simulink model "Control_Law_For_Clay"  (R2020b)
settings: Solver=ode45  StartTime=0.0  StopTime=tsim  RelTol=1e-9
undefined symbols (not defined in the file): fric_mod, g_n, Jm, Jp, K, KcRa, Km, L_n, lambda_n, M_n, N_n, switch_law, T_ba_n, x0
libraries: simulink_extras x3, simulink x1
settings Model: Creator=domin  LastModifiedBy=domin
settings SolverCC: ZeroCrossAlgorithm=Adaptive
settings DebuggingCC: IgnoredZcDiagnostic=none

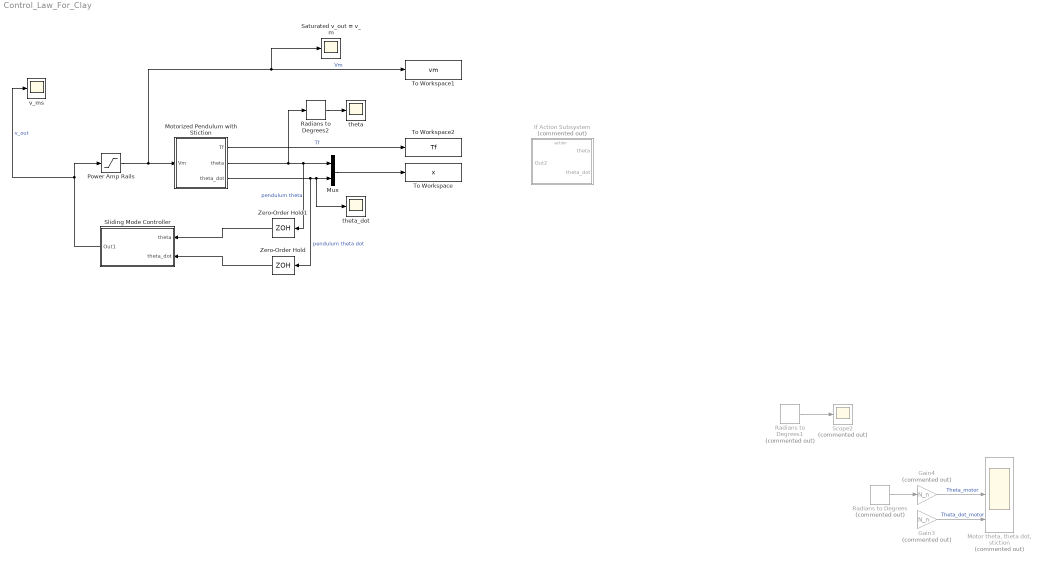
== system Control_Law_For_Clay ==
  Gain3 : Gain  Commented=on  Gain=N_n
  Gain4 : Gain  Commented=on  Gain=N_n
  If Action Subsystem : Subsystem  Commented=on  TreatAsAtomicUnit=on
  "Motor theta, theta dot, stiction" : Scope  Commented=on  NumInputPorts=3
  Motorized Pendulum with Stiction : Subsystem
  Mux : Mux  Inputs=2
  Power Amp Rails : Saturate  UpperLimit=15  LowerLimit=-15
  Radians to Degrees : simulink_extras/Transformations/Radians to Degrees  Commented=on
  Radians to Degrees1 : simulink_extras/Transformations/Radians to Degrees  Commented=on
  Radians to Degrees2 : simulink_extras/Transformations/Radians to Degrees
  Saturated v_out = v_m : Scope
  Scope2 : Scope  Commented=on
  Sliding Mode Controller : Subsystem
  To Workspace : ToWorkspace  VariableName=x  SampleTime=-1
  To Workspace1 : ToWorkspace  VariableName=vm
  To Workspace2 : ToWorkspace  VariableName=Tf  SampleTime=-1
  Zero-Order Hold : ZeroOrderHold  SampleTime=1/100
  Zero-Order Hold1 : ZeroOrderHold  SampleTime=1/100
  theta : Scope
  theta_dot : Scope
  v_ms : Scope
  wires:
  Mux/1 -> To Workspace/1
  Power Amp Rails/1 -> Saturated v_out = v_m/1, To Workspace1/1, Motorized Pendulum with Stiction/1(Vm)  "Vm"
  Motorized Pendulum with Stiction/3(theta_dot) -> Zero-Order Hold/1, theta_dot/1, Mux/2  "pendulum theta dot"
  Motorized Pendulum with Stiction/2(theta) -> Zero-Order Hold1/1, Mux/1, Radians to Degrees2/1  "pendulum theta"
  Radians to Degrees1/1 -> Scope2/1
  Gain4/1 -> "Motor theta, theta dot, stiction"/2  "Theta_motor"
  Radians to Degrees/1 -> Gain4/1
  Gain3/1 -> "Motor theta, theta dot, stiction"/3  "Theta_dot_motor"
  Motorized Pendulum with Stiction/1(Tf) -> To Workspace2/1  "Tf"
  Radians to Degrees2/1 -> theta/1
  Zero-Order Hold1/1 -> Sliding Mode Controller/1(theta)
  Zero-Order Hold/1 -> Sliding Mode Controller/2(theta_dot)
  Sliding Mode Controller/1(Out1) -> v_ms/1, Power Amp Rails/1  "v_out"

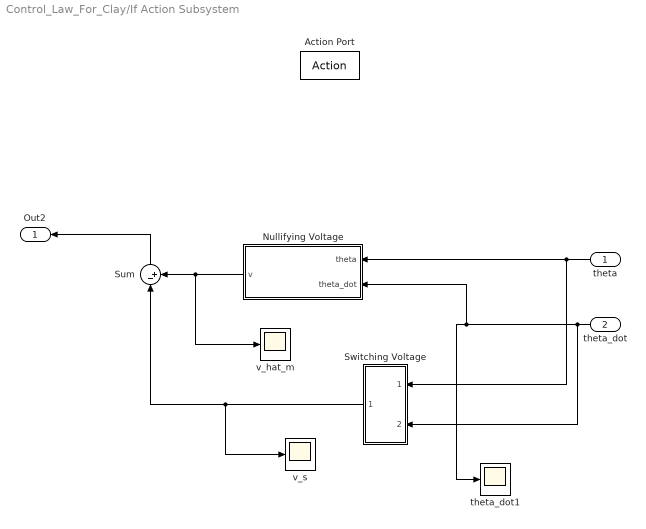
== system Control_Law_For_Clay/If Action Subsystem ==
  theta : Inport
  theta_dot : Inport  Port=2
  Action Port : ActionPort
  Nullifying Voltage : MATLAB Function  TreatAsAtomicUnit=on
  Sum : Sum  Inputs=|-+
  Switching Voltage : Subsystem
  theta_dot1 : Scope
  v_hat_m : Scope
  v_s : Scope
  Out2 : Outport
  wires:
  theta_dot/1 -> Switching Voltage/2(theta_dot), theta_dot1/1, Nullifying Voltage/2(theta_dot)
  theta/1 -> Switching Voltage/1(theta), Nullifying Voltage/1(theta)
  Switching Voltage/1(Out1) -> v_s/1, Sum/1
  Sum/1 -> Out2/1
  Nullifying Voltage/1(v) -> v_hat_m/1, Sum/2

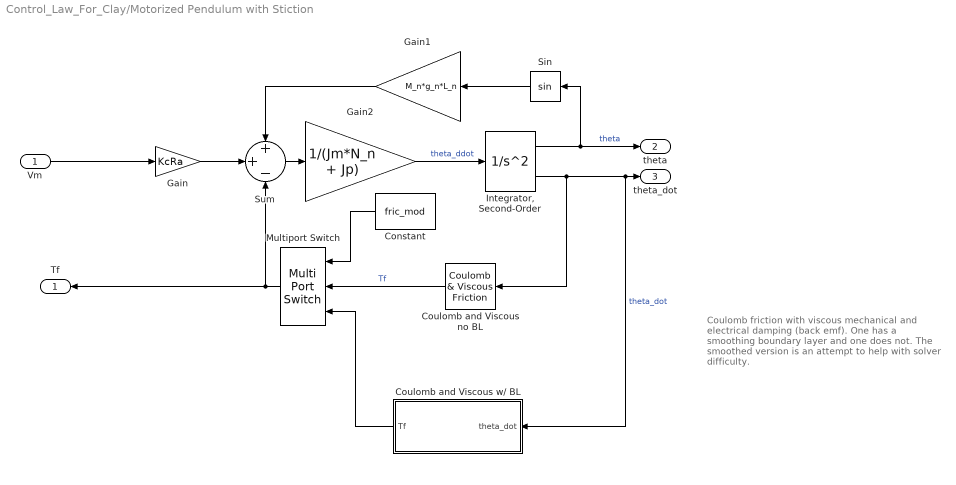
== system Control_Law_For_Clay/Motorized Pendulum with Stiction ==
  note: Coulomb friction with viscous mechanical
      | and electrical damping (back emf). One has a
      | smoothing boundary layer and one does not.
      | The smoothed version is an attempt to help with
      | solver difficulty.
  Vm : Inport
  Constant : Constant  Value=fric_mod
  Coulomb and Viscous no BL : simulink/Discontinuities/Coulomb & Viscous Friction  offset=T_ba_n  gain=N_n*KcRa/Km
  Coulomb and Viscous w/ BL : MATLAB Function  TreatAsAtomicUnit=on
  Gain : Gain  Gain=KcRa
  Gain1 : Gain  Gain=M_n*g_n*L_n
  Gain2 : Gain  Gain=1/(Jm*N_n + Jp)
  "Integrator, Second-Order" : SecondOrderIntegrator  ICX=x0(1)  ICDXDT=x0(2)  ZeroCross=off
  Multiport Switch : MultiPortSwitch  Inputs=2
  Sin : Trigonometry
  Sum : Sum  Inputs=++-
  Tf : Outport
  theta : Outport  Port=2
  theta_dot : Outport  Port=3
  wires:
  Gain2/1 -> "Integrator, Second-Order"/1  "theta_ddot"
  Sin/1 -> Gain1/1
  "Integrator, Second-Order"/2 -> Coulomb and Viscous w/ BL/1(theta_dot), theta_dot/1, Coulomb and Viscous no BL/1  "theta_dot"
  "Integrator, Second-Order"/1 -> Sin/1, theta/1  "theta"
  Gain1/1 -> Sum/1
  Sum/1 -> Gain2/1
  Vm/1 -> Gain/1
  Gain/1 -> Sum/2
  Constant/1 -> Multiport Switch/1
  Multiport Switch/1 -> Tf/1, Sum/3
  Coulomb and Viscous w/ BL/1(Tf) -> Multiport Switch/3
  Coulomb and Viscous no BL/1 -> Multiport Switch/2  "Tf"

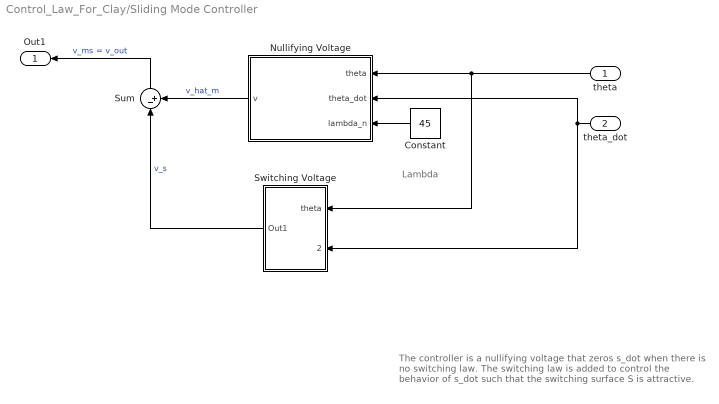
== system Control_Law_For_Clay/Sliding Mode Controller ==
  note: The controller is a nullifying voltage that zeros s_dot
      | when there is no switching law. The switching law is added
      | to control the behavior of s_dot such that the switching surface
      | S is attractive.
  note: Lambda
  theta : Inport
  theta_dot : Inport  Port=2
  Constant : Constant  Value=45
  Nullifying Voltage : MATLAB Function  TreatAsAtomicUnit=on
  Sum : Sum  Inputs=|-+
  Switching Voltage : Subsystem
  Out1 : Outport
  wires:
  Nullifying Voltage/1(v) -> Sum/2  "v_hat_m"
  Sum/1 -> Out1/1  "v_ms = v_out"
  theta/1 -> Switching Voltage/1(theta), Nullifying Voltage/1(theta)
  theta_dot/1 -> Switching Voltage/2(theta_dot), Nullifying Voltage/2(theta_dot)
  Switching Voltage/1(Out1) -> Sum/1  "v_s"
  Constant/1 -> Nullifying Voltage/3(lambda_n)

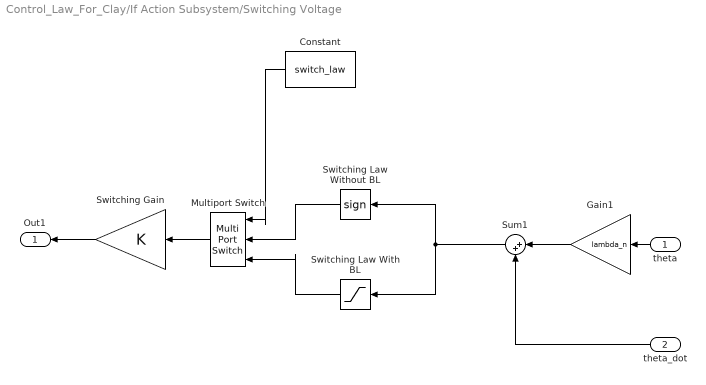
== system Control_Law_For_Clay/If Action Subsystem/Switching Voltage ==
  theta : Inport
  theta_dot : Inport  Port=2
  Constant : Constant  Value=switch_law
  Gain1 : Gain  Gain=lambda_n
  Multiport Switch : MultiPortSwitch  Inputs=2
  Sum1 : Sum  Inputs=|++
  Switching Gain : Gain  Gain=K
  Switching Law With BL : Saturate  UpperLimit=1  LowerLimit=-1
  Switching Law Without BL : Signum
  Out1 : Outport
  wires:
  Gain1/1 -> Sum1/1
  theta/1 -> Gain1/1
  Switching Gain/1 -> Out1/1
  Sum1/1 -> Switching Law With BL/1, Switching Law Without BL/1
  theta_dot/1 -> Sum1/2
  Constant/1 -> Multiport Switch/1
  Multiport Switch/1 -> Switching Gain/1
  Switching Law Without BL/1 -> Multiport Switch/2
  Switching Law With BL/1 -> Multiport Switch/3

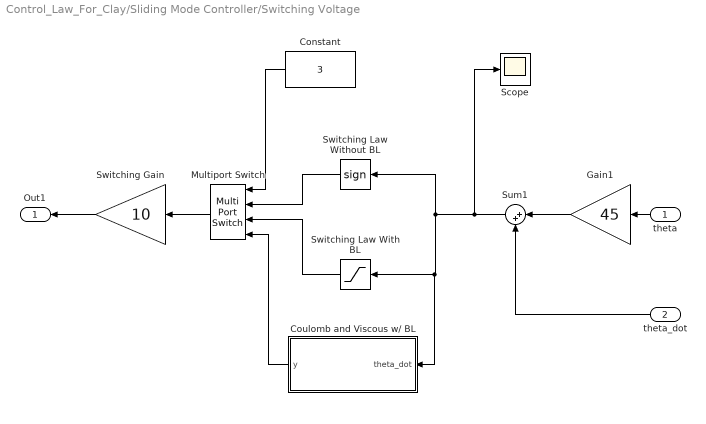
== system Control_Law_For_Clay/Sliding Mode Controller/Switching Voltage ==
  theta : Inport
  theta_dot : Inport  Port=2
  Constant : Constant  Value=3
  Coulomb and Viscous w/ BL : MATLAB Function  TreatAsAtomicUnit=on
  Gain1 : Gain  Gain=45
  Multiport Switch : MultiPortSwitch
  Scope : Scope
  Sum1 : Sum  Inputs=|++
  Switching Gain : Gain  Gain=10
  Switching Law With BL : Saturate  UpperLimit=1  LowerLimit=-1
  Switching Law Without BL : Signum
  Out1 : Outport
  wires:
  Gain1/1 -> Sum1/1
  theta/1 -> Gain1/1
  Switching Gain/1 -> Out1/1
  Sum1/1 -> Scope/1, Coulomb and Viscous w/ BL/1(theta_dot), Switching Law With BL/1, Switching Law Without BL/1
  theta_dot/1 -> Sum1/2
  Constant/1 -> Multiport Switch/1
  Multiport Switch/1 -> Switching Gain/1
  Switching Law Without BL/1 -> Multiport Switch/2
  Switching Law With BL/1 -> Multiport Switch/3
  Coulomb and Viscous w/ BL/1(y) -> Multiport Switch/4

== matlab function Control_Law_For_Clay/Motorized Pendulum with Stiction/Coulomb and Viscous w// BL ==
  data: theta_dot input; Tf output; Km parameter; KcRa parameter; N_n parameter; T_ba_n parameter
function Tf = fcn(theta_dot, Km,  KcRa, N_n, T_ba_n)

Tf = N_n*KcRa/Km*theta_dot + T_ba_n*erf(1e6*theta_dot);

== matlab function Control_Law_For_Clay/Sliding Mode Controller/Nullifying Voltage ==
  data: theta input; theta_dot input; v output; K parameter; lambda_n input
function v = fcn(theta, theta_dot, K, lambda_n)


v = 0.3501*theta_dot - 1.0684*sign(theta_dot) - 0.6600*sin(theta_dot)...
    - 0.1144*lambda_n*theta_dot;

== matlab function Control_Law_For_Clay/If Action Subsystem/Nullifying Voltage ==
  data: theta input; theta_dot input; v output; lambda_n parameter; K parameter
function v = fcn(theta, theta_dot, lambda_n, K)


% v = 0.3401*theta_dot - 1.0684*sign(theta_dot) - 0.6600*sin(theta)...
%     - 0.1144*lambda_n*theta_dot;

v = 0.3501*theta_dot - 1.0684*sign(theta_dot) - 0.6600*sin(theta_dot)...
    - 0.1144*lambda_n*theta_dot;

== matlab function Control_Law_For_Clay/Sliding Mode Controller/Switching Voltage/Coulomb and Viscous w// BL ==
  data: theta_dot input; y output; err_fnc_coeff parameter
function y = fcn(theta_dot, err_fnc_coeff)

y = erf(0.9*theta_dot);
